simulink model "stm32_buck_vmc_host_read"  (R2022a)
settings: Solver=VariableStepAuto  StartTime=0.0  StopTime=inf  RelTol=1e-3
libraries: instrumentseriallib x2
settings Model: Creator=rkandur  LastModifiedBy=User
settings SolverCC: AlgebraicLoopSolver=TrustRegion  MaxZcPerStep=1
settings DebuggingCC: ParameterPrecisionLossMsg=none  UnconnectedInputMsg=warning  UnconnectedOutputMsg=warning  UnconnectedLineMsg=warning  SFMachineParentedDataDiag=warning
settings RTWCC: DLArmComputeVersion=19.05

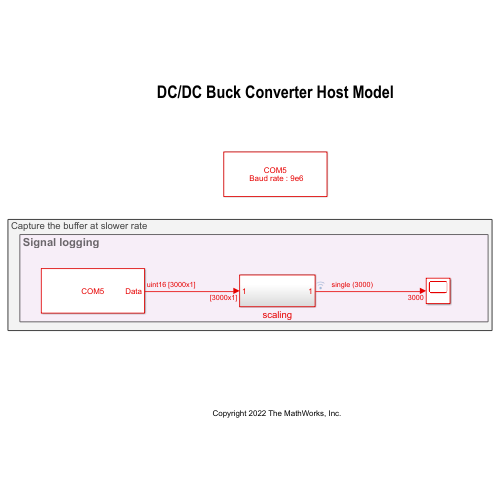
[thumbnail: Simulink's stored preview of the top-level diagram]
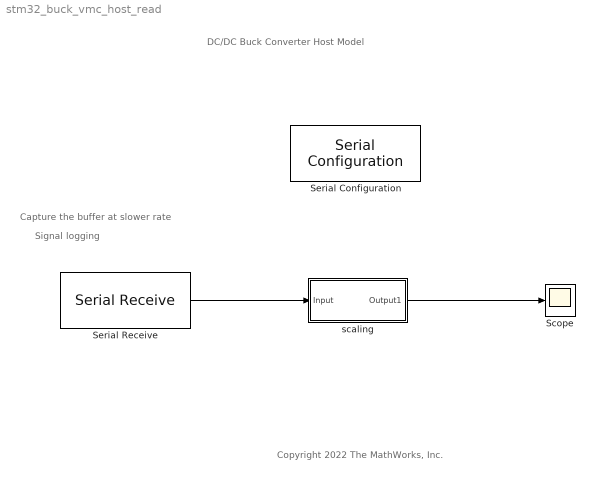
== system stm32_buck_vmc_host_read ==
  note: Capture the buffer at slower rate
  note: Copyright 2022 The MathWorks, Inc.
  note: DC/DC Buck Converter Host Model
  note: Signal logging
  Scope : Scope
  Serial Configuration : instrumentseriallib/Serial Configuration  Priority=-200000  PortSel=COM5  Port=COM5  ComPort=COM5  BaudRate=9e6  DataBits=8  Parity=none  StopBits=1  ByteOrder=little-endian  FlowControl=none  Timeout=1  SimulateUsing=Interpreted execution  BlockInModel=on  aMode=1
      settings: SourceProductBaseCode=OT,IC,MT
  Serial Receive : instrumentseriallib/Serial Receive  PortSel=COM5  Port=COM5  ComPort=COM5  DataType=uint16  SaveDataType=uint8  ToggleHeader=on  Header='SS'  ToggleTerminator=on  Terminator=Custom terminator  CustomTerminator='EE'  InputFormat=Row major  ToggleDataSize=on  DataSize=[3000]  EnableBlockingMode=on  ActionDataUnavailable=Output last received value  ActionWhenDataUnavailable=Output last received value  CustomValue=0  SampleTime=0.06  SimulateUsing=Interpreted execution  BlockInModel=on  aMode=1
      settings: SourceProductBaseCode=OT,IC,MT
  scaling : Subsystem
  wires:
  Serial Receive/1 -> scaling/1(Input)
  scaling/1(Output1) -> Scope/1

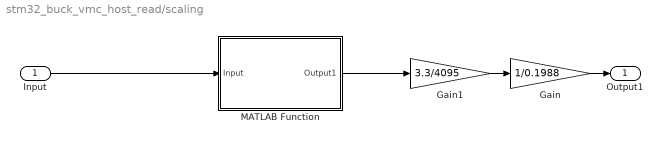
== system stm32_buck_vmc_host_read/scaling ==
  Input : Inport
  Gain : Gain  Gain=1/0.1988
  Gain1 : Gain  Gain=3.3/4095  OutDataTypeStr=single
  MATLAB Function : MATLAB Function  TreatAsAtomicUnit=on
  Output1 : Outport  VectorParamsAs1DForOutWhenUnconnected=off
  wires:
  Input/1 -> MATLAB Function/1(Input)
  MATLAB Function/1(Output1) -> Gain1/1
  Gain/1 -> Output1/1
  Gain1/1 -> Gain/1

== matlab function stm32_buck_vmc_host_read/scaling/MATLAB Function ==
  data: Output1 output; Input input
function Output1  = unBuf(Input)

Output1 = Input(:, 1);
end
